simulink model "ex2"  (R2020b)
settings: Solver=VariableStepAuto  StartTime=0.0  StopTime=2  RelTol=1e-3
InitFcn:
  | A = [-10 1; 0.02 -2];
  | B = [0;2];
  | Q = eye(2);
  | R = 1;
  | 
  | K = lqr(A,B,Q,R);
  | 
  | A1 = [10 1; 1 10];
  | A2 = [20 2; 2 20];
  | kappa = 1;
  | 
  | x0 = rand(2,1);
libraries: ctrlSharedLib x1
settings Model: Creator=toetotoe  LastModifiedBy=toetotoe

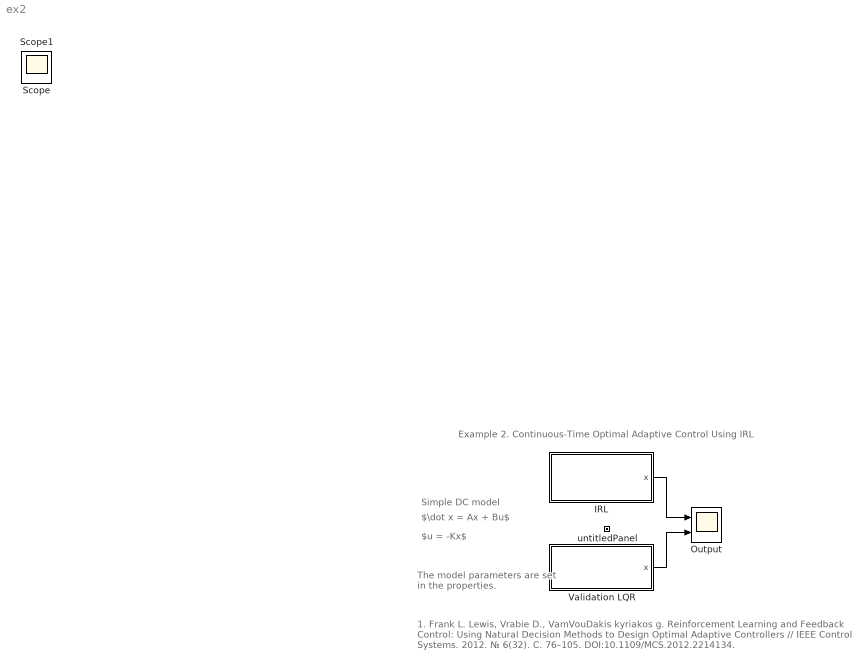
== system ex2 ==
  note: The model parameters
      | are set in the properties.
  note: 1. Frank L. Lewis, Vrabie D., VamVouDakis kyriakos g. Reinforcement Learning and Feedback Control: Using Natural Decision Methods to Design Optimal Adaptive Controllers // IEEE Control Systems. 2012. № 6(32). С. 76–105. DOI:10.1109/MCS.2012.2214134.
  note: $u = -Kx$
  note: Simple DC model
  note: $\dot x = Ax + Bu$
  note: Example 2. Continuous-Time Optimal Adaptive Control Using IRL
  IRL : Subsystem
  Output : Scope  NumInputPorts=2
  Validation LQR : Subsystem
  untitledPanel : Subsystem  Tag=HiddenForWebPanel  IsWebBlockPanel=on
  Scope : Scope
  Scope1 : Scope
  wires:
  Validation LQR/1(x) -> Output/2
  IRL/1(x) -> Output/1

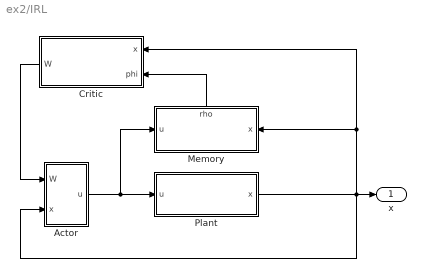
== system ex2/IRL ==
  Actor : Subsystem
  Critic : Subsystem
  Memory : Subsystem
      settings: PortSchema="{\"entries\":[{\"content\":{\"sides\":[{\"content\":{\"connectorIds\":[\"In1\"]},\"type\":\"ConnectorPlacement.EquallySpacedRectSide\",\"uuid\":\"a5ff65ef-635e-4f46-88b6-897d9eca60b5\"},{\"content\":{\"connectorIds\":[\"In2\"],\"side\":\"RIGHT\"},\"type\":\"ConnectorPlacement.EquallySpacedRectSide\",\"uuid\":\"e2705bc7-1aad-44cb-b2c9-3c4f163857d1\"},{\"content\":{\"connectorIds\":[\"Out1\"],\"side\":\"TOP\"},\"type\":\"ConnectorPlacement.EquallySpacedRectSide\",\"uuid\":\"be6bf656-f908-4f0d-834e-0ce759f025a5\"},{\"content\":{\"connectorIds\":[],\"side\":\"HIDDEN\"},\"type\":\"ConnectorPlacement.EquallySpacedRectSide\",\"uuid\":\"e57eeeaf-f06a-4fc7-959d-0f4b982e6bfd\"}]},\"type\":\"ConnectorPlacement.EquallySpacedConnector\",\"uuid\":\"503d1bbf-e0b5-4dcb-9a4d-7ac319c614b6\"}],\"packageUris\":[\"http://schema.mathworks.com/mf0/Connector/R2020b\"],\"version\":\"1.0\"}"
  Plant : Subsystem
  x : Outport
  wires:
  Actor/1(u) -> Memory/1(u), Plant/1(u)
  Memory/1(rho) -> Critic/2(phi)
  Critic/1(W) -> Actor/1(W)
  Plant/1(x) -> Actor/2(x), x/1, Critic/1(x), Memory/2(x)

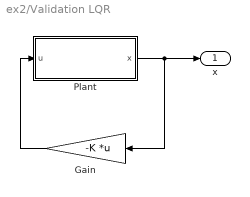
== system ex2/Validation LQR ==
  Gain : Gain  Gain=-K  Multiplication=Matrix(K*u) (u vector)
  Plant : Subsystem
  x : Outport
  wires:
  Gain/1 -> Plant/1(u)
  Plant/1(x) -> Gain/1, x/1

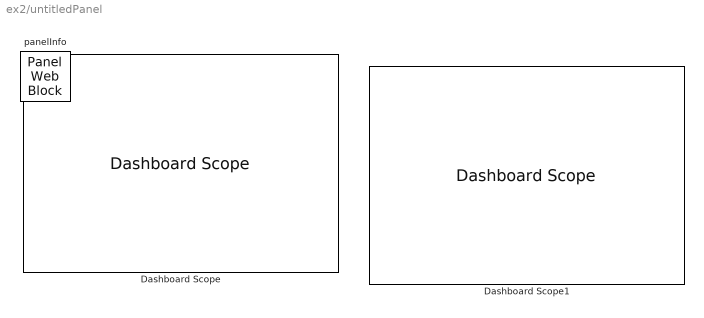
== system ex2/untitledPanel ==
  Dashboard Scope : DashboardScope  Tag=HiddenForWebPanel  PanelInfo="{\"panelId\":\"panelId-d583a1d5-43fa-4411-94d7-e392976298f4\",\"type\":\"panelChild\",\"version\":\"2019b\",\"zIndex\":1500002}"
  Dashboard Scope1 : DashboardScope  Tag=HiddenForWebPanel  PanelInfo="{\"panelId\":\"panelId-d583a1d5-43fa-4411-94d7-e392976298f4\",\"type\":\"panelChild\",\"version\":\"2019b\",\"zIndex\":1500004}"
  panelInfo : PanelWebBlock  Tag=HiddenForWebPanel  PanelInfo="{\"compacted\":true,\"height\":270,\"left\":301,\"name\":\"untitledPanel\",\"panelId\":\"panelId-d583a1d5-43fa-4411-94d7-e392976298f4\",\"top\":152,\"type\":\"panel\",\"version\":\"2019b\",\"visible\":true,\"width\":701,\"zIndex\":1500002}"  PanelSnapshot=<binary blob, 19560 chars, not shown>

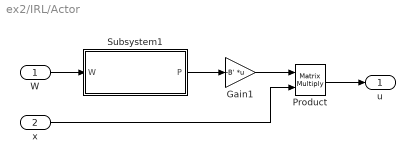
== system ex2/IRL/Actor ==
  W : Inport
  x : Inport  Port=2
  Gain1 : Gain  Gain=-B'  Multiplication=Matrix(K*u)
  Product : Product  Multiplication=Matrix(*)
  Subsystem1 : Subsystem
  u : Outport
  wires:
  W/1 -> Subsystem1/1(W)
  Subsystem1/1(P) -> Gain1/1
  x/1 -> Product/2
  Product/1 -> u/1
  Gain1/1 -> Product/1

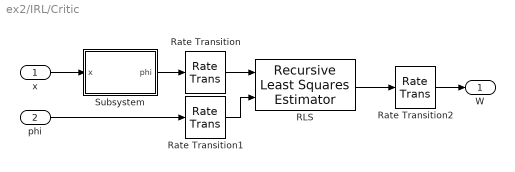
== system ex2/IRL/Critic ==
  x : Inport
  phi : Inport  Port=2
  RLS : ctrlSharedLib/Recursive Least Squares Estimator  InitialEstimateSource=None  InitialParameterData=3  P0=1e4  InitialRegressors=0  InitialOutputs=0  History=Infinite  WindowLength=200  EstimationMethod=Forgetting Factor  AdaptationParameter=1  HasTimeVaryingAdaptationParameter=off  NormalizationBias=eps  OutputError=off  OutputP=off  AddEnablePort=off  InputProcessing=Sample-based  Ts=0.04
      settings: SourceProductBaseCode=CT,ID
  Rate Transition : RateTransition  OutPortSampleTime=0.04
  Rate Transition1 : RateTransition  OutPortSampleTime=0.04
  Rate Transition2 : RateTransition  OutPortSampleTime=0.2
  Subsystem : Subsystem
  W : Outport
  wires:
  phi/1 -> Rate Transition1/1
  x/1 -> Subsystem/1(x)
  Rate Transition2/1 -> W/1
  RLS/1 -> Rate Transition2/1
  Subsystem/1(phi) -> Rate Transition/1
  Rate Transition1/1 -> RLS/2
  Rate Transition/1 -> RLS/1

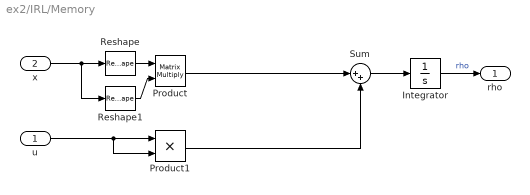
== system ex2/IRL/Memory ==
  u : Inport
  x : Inport  Port=2
  Integrator : Integrator
  Product : Product  Multiplication=Matrix(*)
  Product1 : Product
  Reshape : Reshape  OutputDimensionality=Row vector (2-D)
  Reshape1 : Reshape  OutputDimensionality=Column vector (2-D)
  Sum : Sum  Inputs=|++
  rho : Outport
  wires:
  Integrator/1 -> rho/1  "rho"
  Reshape/1 -> Product/1
  x/1 -> Reshape1/1, Reshape/1
  Reshape1/1 -> Product/2
  Product/1 -> Sum/1
  Product1/1 -> Sum/2
  Sum/1 -> Integrator/1
  u/1 -> Product1/2, Product1/1

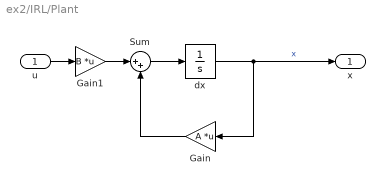
== system ex2/IRL/Plant ==
  u : Inport
  Gain : Gain  Gain=A  Multiplication=Matrix(K*u)
  Gain1 : Gain  Gain=B  Multiplication=Matrix(K*u)
  Sum : Sum  Inputs=|++
  dx : Integrator  InitialCondition=x0
  x : Outport
  wires:
  dx/1 -> Gain/1, x/1  "x"
  Sum/1 -> dx/1
  Gain/1 -> Sum/2
  u/1 -> Gain1/1
  Gain1/1 -> Sum/1

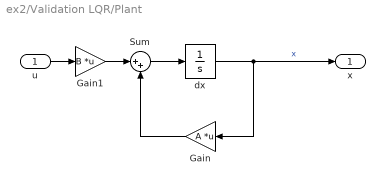
== system ex2/Validation LQR/Plant ==
  u : Inport
  Gain : Gain  Gain=A  Multiplication=Matrix(K*u)
  Gain1 : Gain  Gain=B  Multiplication=Matrix(K*u)
  Sum : Sum  Inputs=|++
  dx : Integrator  InitialCondition=x0
  x : Outport
  wires:
  dx/1 -> Gain/1, x/1  "x"
  Sum/1 -> dx/1
  Gain/1 -> Sum/2
  u/1 -> Gain1/1
  Gain1/1 -> Sum/1

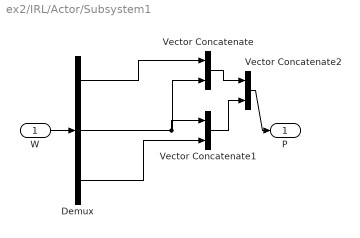
== system ex2/IRL/Actor/Subsystem1 ==
  W : Inport
  Demux : Demux  Outputs=3
  Vector Concatenate : Concatenate
  Vector Concatenate1 : Concatenate
  Vector Concatenate2 : Concatenate  Mode=Multidimensional array  ConcatenateDimension=2
  P : Outport
  wires:
  W/1 -> Demux/1
  Vector Concatenate1/1 -> Vector Concatenate2/2
  Vector Concatenate/1 -> Vector Concatenate2/1
  Vector Concatenate2/1 -> P/1
  Demux/1 -> Vector Concatenate/1
  Demux/2 -> Vector Concatenate1/1, Vector Concatenate/2
  Demux/3 -> Vector Concatenate1/2

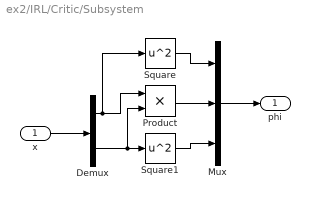
== system ex2/IRL/Critic/Subsystem ==
  x : Inport
  Demux : Demux  Outputs=2
  Mux : Mux  Inputs=3
  Product : Product
  Square : Math  Operator=square  SaturateOnIntegerOverflow=on
  Square1 : Math  Operator=square  SaturateOnIntegerOverflow=on
  phi : Outport
  wires:
  Demux/2 -> Square1/1, Product/2
  Square1/1 -> Mux/3
  Product/1 -> Mux/2
  x/1 -> Demux/1
  Square/1 -> Mux/1
  Demux/1 -> Square/1, Product/1
  Mux/1 -> phi/1
